simulink model "bloc_inteligent"  (R2026a)
settings: Solver=VariableStepAuto  StopTime=60
settings Model: Creator=Alex  LastModifiedBy=Alex

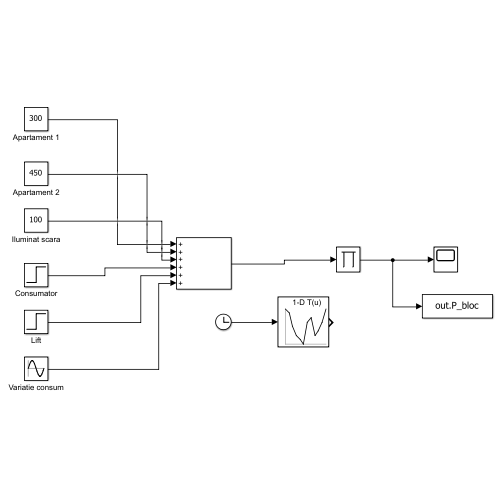
[thumbnail: Simulink's stored preview of the top-level diagram]
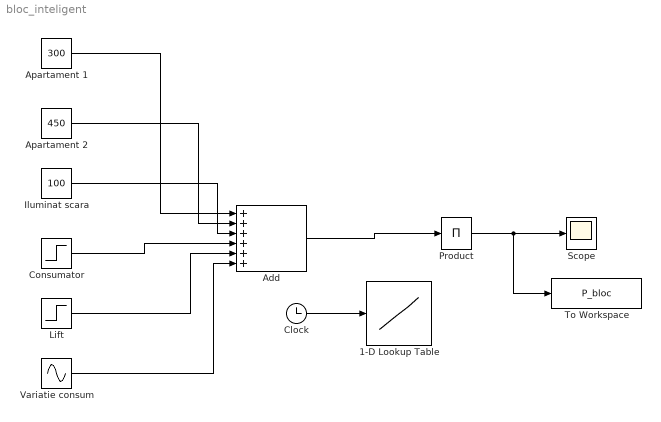
== system bloc_inteligent ==
  1-D Lookup Table : Lookup_n-D  NumberOfTableDimensions=1  BreakpointsForDimension1=[1 2 3 4 5 6 7 8 9 10 11 12]  Table=[1.3 1.25 1.1 1.0 0.95 0.9 1.15 1.2 1.0 1.05 1.15 1.3]  InternalRulePriority=Speed  RndMeth=Simplest
  Add : Sum  Inputs=++++++
  Apartament 1 : Constant  Value=300
  Apartament 2 : Constant  Value=450
  Clock : Clock
  Consumator : Step  Time=20  FinalValue=400  SampleTime=0
  Iluminat scara : Constant  Value=100
  Lift : Step  Time=50  FinalValue=600  SampleTime=0
  Product : Product  Inputs=1
  Scope : Scope
      settings: ActiveDisplayYMinimum=-43466.705774410249  ActiveDisplayYMaximum=109693.12428445267
  To Workspace : ToWorkspace  VariableName=P_bloc  SampleTime=-1
  Variatie consum : Sin  Amplitude=50  Bias=100  Frequency=0.1  SampleTime=0
  wires:
  Clock/1 -> 1-D Lookup Table/1
  Apartament 1/1 -> Add/1
  Apartament 2/1 -> Add/2
  Iluminat scara/1 -> Add/3
  Consumator/1 -> Add/4
  Lift/1 -> Add/5
  Variatie consum/1 -> Add/6
  Add/1 -> Product/1
  Product/1 -> To Workspace/1, Scope/1
